simulink model "linefollowing"  (R2020a)
settings: Solver=FixedStepDiscrete  StartTime=0.0  StopTime=10.0  FixedStep=0.01  RelTol=1e-3
undefined symbols (not defined in the file or in its folder): motorIp, motorSp
libraries: mobileRoboticsTrainingLib x5
settings Model: Creator=Navyasree  LastModifiedBy=Navyasree

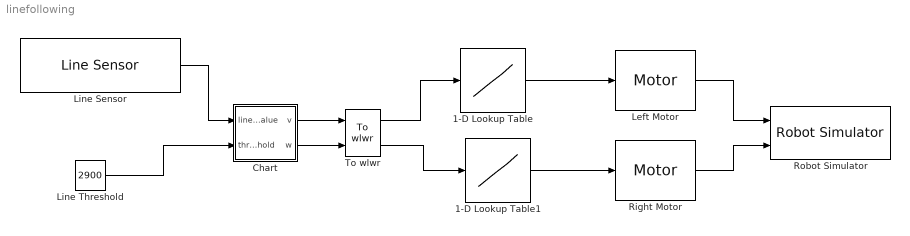
== system linefollowing ==
  1-D Lookup Table : Lookup_n-D  NumberOfTableDimensions=1  BreakpointsForDimension1=motorSp  Table=motorIp  InternalRulePriority=Speed  RndMeth=Simplest  InputSameDT=on
  1-D Lookup Table1 : Lookup_n-D  NumberOfTableDimensions=1  BreakpointsForDimension1=motorSp  Table=motorIp  InternalRulePriority=Speed  RndMeth=Simplest  InputSameDT=on
  Chart : Stateflow chart  TreatAsAtomicUnit=on
  Left Motor : mobileRoboticsTrainingLib/Motor  motorPlant=wheelMotorModel  sensorType=Speed
      settings: SourceProductName=Mobile Robotics Training Library
  Line Sensor : mobileRoboticsTrainingLib/Line Sensor  mapVariable=mapForSim  envVal=2850  lineVal=2950  sensOff=[0.01 0]
      settings: SourceProductName=Mobile Robotics Training Library
  Line Threshold : Constant  Value=2900
  Right Motor : mobileRoboticsTrainingLib/Motor  motorPlant=wheelMotorModel  sensorType=Speed
      settings: SourceProductName=Mobile Robotics Training Library
  Robot Simulator : mobileRoboticsTrainingLib/Robot Simulator  Priority=99  mapVar=mapForSim  startX=0.6119  startY=1.3086  startTheta=0  axleLength=axleLength  wheelR=wheelR
  To wlwr : mobileRoboticsTrainingLib/To wlwr  axleLength=0.1  wheelR=0.05
  wires:
  Line Threshold/1 -> Chart/2(threshold)
  Line Sensor/1 -> Chart/1(linevalue)
  Chart/1(v) -> To wlwr/1
  Chart/2(w) -> To wlwr/2
  To wlwr/1 -> 1-D Lookup Table/1
  To wlwr/2 -> 1-D Lookup Table1/1
  1-D Lookup Table/1 -> Left Motor/1
  1-D Lookup Table1/1 -> Right Motor/1
  Left Motor/1 -> Robot Simulator/1
  Right Motor/1 -> Robot Simulator/2

== stateflow chart linefollowing/Chart ==
  state GoLeft
    v=0.05
    w=1
  state GoRight
    v=0.05
    w=-1
  (default) -> GoLeft
  GoLeft -> GoRight : [linevalue<threshold]
  GoRight -> GoLeft : [linevalue>threshold]
  data: linevalue input; threshold input; v output; w output
